simulink model "back_project"  (R2020b)
settings: Solver=VariableStepAuto  StartTime=0.0  StopTime=10.0  RelTol=1e-3
model workspace: external: MAT-File /Users/tomoffat/Documents/final_year_coursework/fyp/blender/sar_consts.mat (data not in the file)
values from neighbouring files (symbols this model uses):
  c = physconst('LightSpeed')    [omegak.m]    (also in sar_consts.mat = 299792458; sar_script_ref.m)
  crossRangeResolution = 3    [sar_consts.mat]    (also in sar_script_ref.m)
  fastTime = [0 8.33333333333e-09 1.66666666667e-08 2.5e-08 3.33333333333e-08 4.16666666667e-08 5e-08 5.83333333333e-08 6.66666666667e-08 7.5e-08 8.33333333333e-08 9.16666666667e-08 ... (2002 elements, 1x2002)]    [sar_consts.mat]    (also in sar_script_ref.m = (0:1/fs:(truncrangesamples-1)/fs))
  fc = 4000000000    [sar_consts.mat]    (also in sar_script_ref.m)
  fs = 120000000    [sar_consts.mat]    (also in sar_script_ref.m)
  prf = 1000    [sar_consts.mat]    (also in sar_script_ref.m)
  speed = 400    [sar_consts.mat]    (also in sar_script_ref.m = 100)
undefined symbols (not defined in the file or in its folder): get, hot, out, physconst
libraries: dspsnks4 x1, phaseddetectlib x1
settings Model: Creator=tomoffat  LastModifiedBy=tomoffat

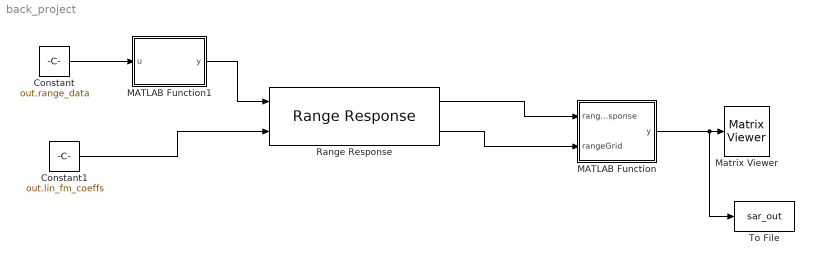
== system back_project ==
  Constant : Constant  Value=out.range_data
  Constant1 : Constant  Value=out.lin_fm_coeffs  VectorParams1D=off
  MATLAB Function : MATLAB Function  TreatAsAtomicUnit=on
  MATLAB Function1 : MATLAB Function  TreatAsAtomicUnit=on
  Matrix Viewer : dspsnks4/Matrix Viewer  ImageParams=off  CMapStr=hot(256)  AxisColorbar=on  AxisParams=off  AxisOrigin=Upper left corner  AxisTickMode=Auto  XTickRange=[0 1]  YTickRange=[0 1]  XLabel=Cross-Range Samples  YLabel=Range Samples  ZLabel=Z-axis  FigPos=get(0,'defaultfigureposition')  AxisZoom=off
      settings: SourceProductBaseCode=DS  YMin=0  YMax=255
  Range Response : phaseddetectlib/Range Response  RangeMethod=Matched filter  PropagationSpeed=physconst( 'lightspeed' )  SampleRateFromInputCheckbox=on  SampleRate=1e6  SweepSlope=1e9  DechirpInput=off  RangeFFTLengthSource=Auto  RangeFFTLength=1024  RangeWindow=None  RangeSidelobeAttenuation=30  CustomRangeWindow=@hamming  ReferenceRangeCentered=on  ReferenceRange=0  MaximumNumInputSamplesSource=Auto  MaximumNumInputSamples=100  SimulateUsing=Interpreted execution
      settings: SourceProductBaseCode=AR
  To File : ToFile  Filename=sar_out  SaveFormat=Timeseries
  wires:
  MATLAB Function/1(y) -> To File/1, Matrix Viewer/1
  Constant1/1 -> Range Response/2
  Range Response/1 -> MATLAB Function/1(rangeResponse)
  Range Response/2 -> MATLAB Function/2(rangeGrid)
  Constant/1 -> MATLAB Function1/1(u)
  MATLAB Function1/1(y) -> Range Response/1

== matlab function back_project/MATLAB Function1 ==
  data: u input; y output
function y = fcn(u)

y = reshape(u, 2002, []);

== matlab function back_project/MATLAB Function ==
  data: rangeResponse input; y output; rangeGrid input; speed parameter; prf parameter; c parameter; fc parameter; fastTime parameter; crossRangeResolution parameter; fs parameter
function y = fcn(rangeResponse, rangeGrid, speed, prf, c, fc, fastTime, crossRangeResolution, fs)
    
    data = zeros(size(rangeResponse));
    azimuthDist = -200:400/1000:200;%azimuth distance
    rangelims = [700 1400];
    crossrangelims = [-10 10];
    rangeIdx =  [find(rangeGrid>rangelims(1), 1) find(rangeGrid<rangelims(2),1,'last')];
    crossrangeIdxStart = find(azimuthDist>crossrangelims(1),1);
    crossrangeIdxStop = find(azimuthDist<crossrangelims(2),1,'last');
    for i= rangeIdx(1):rangeIdx(2)  % Iterate over the range indices
    
        % Using desired cross-range resolution, compute the synthetic aperture
        % length
        lsynth= (c/fc)* (c*fastTime(i)/2)/(2*crossRangeResolution);
        lsar = round(lsynth*length(azimuthDist)/azimuthDist(end)) ;
        % Ensure lsar is an odd number
        lsar = lsar + mod(lsar,2);    
    
        % Construct hanning window for cross-range processing, to suppress the
        % azimuthal side lobes
        hn= hanning(lsar).';
        % Iterate over the cross-range indices
        for j = crossrangeIdxStart:crossrangeIdxStop 
            % azimuth distance in x direction over cross-range indices
            posx = azimuthDist(j);
            % range in y-direction over range indices
            posy= c*fastTime(i)/2;
            % initializing count to zero
            count= 0;
            % Iterate over the synthetic aperture
            for k= j-lsar/2 +1:j+ lsar/2 
                % Time delay for each of range and cross-range indices
                td= sqrt((azimuthDist(k)- posx)^2 + posy^2)*2/c;
                cell= round(td*fs) +1 ;
                signal = rangeResponse(cell,k);
                count= count + hn(k -(j-lsar/2))*signal *exp(1j*2*pi*fc*(td));
            end
            % Processed data at each of range and cross-range indices
            data(i,j)= count;
        end
    
    end
y = data;
